simulink model "MeasModelCompare_lambda"  (Simulink 7.9)
settings: Solver=ode45  StartTime=0.0  StopTime=10.0  RelTol=1e-5  AbsTol=1e-5
values from neighbouring files (symbols this model uses):
  fake_lambda_cyl = [ones(stepTime,1); 0.8*ones(numel(FuelStep.t)-stepTime,1)]    [Init_Project1.m]
  tau_d_bc = 0.05    [Init_Project1.m]
  tau_lambda = 0.21    [Init_Project1.m]
settings Model: Creator=oberg  LastModifiedBy=nicgr354  ExtModeAutoUpdateStatusClock=off
settings DataIOCC: SignalLoggingName=sigsOut
settings DebuggingCC: ConsistencyChecking=warning  SaveWithParameterizedLinksMsg=none  SignalResolutionControl=TryResolveAllWithWarning  SolverPrmCheckMsg=none  MultiTaskDSMMsg=warning  MultiTaskCondExecSysMsg=none  StrictBusMsg=None
settings HardwareCC: TargetUnknown=on
settings RTWCC: IncludeERTFirstTime=on
settings CodeAppCC: CustomSymbolStrType=$N$R$M_T
settings GRTTargetCC: CodeReplacementLibrary=None  CombineOutputUpdateFcns=off  CPPClassGenCompliant=on  GRTInterface=on

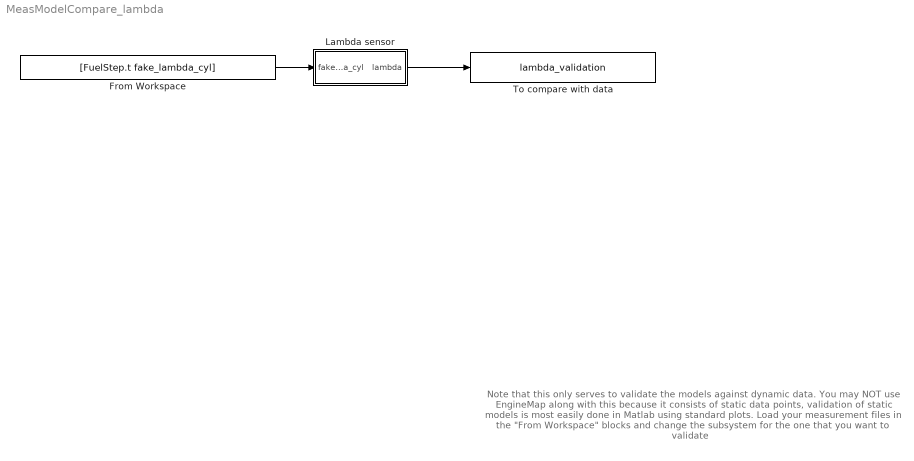
== system MeasModelCompare_lambda ==
  note: Note that this only serves to validate the models against dynamic data.
      | You may NOT use EngineMap along with this because it consists of static data points,
      | validation of static models is most easily done in Matlab using standard plots.
      |
      | Load your measurement files in the "From Workspace" blocks
      | and change the subsystem for the one that you want to validate
  From Workspace : FromWorkspace  VariableName=[FuelStep.t fake_lambda_cyl]  SampleTime=0
  Lambda sensor : Subsystem
  To compare with data : ToWorkspace  VariableName=lambda_validation  SampleTime=-1  SaveFormat=Structure With Time
  wires:
  Lambda sensor/1(lambda) -> To compare with data/1
  From Workspace/1 -> Lambda sensor/1(fake_lambda_cyl)

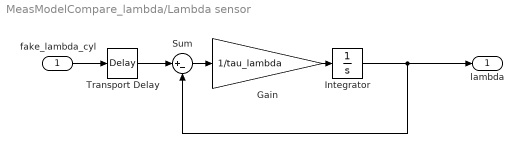
== system MeasModelCompare_lambda/Lambda sensor ==
  fake_lambda_cyl : Inport
  Gain : Gain  Gain=1/tau_lambda
  Integrator : Integrator  InitialCondition=fake_lambda_cyl(1)
  Sum : Sum  Inputs=|+-  SaturateOnIntegerOverflow=on
  Transport Delay : TransportDelay  DelayTime=tau_d_bc  InitialOutput=1
  lambda : Outport
  wires:
  fake_lambda_cyl/1 -> Transport Delay/1
  Transport Delay/1 -> Sum/1
  Integrator/1 -> lambda/1, Sum/2
  Sum/1 -> Gain/1
  Gain/1 -> Integrator/1
